simulink model "simulink_cordic_cart2pol_model"  (R2018a)
settings: Solver=FixedStepDiscrete  StartTime=0.0  StopTime=inf  RelTol=1e-3
undefined symbols (not defined in the file or in its folder): cordic_table, gap, niter, pipe, x_in, y_in
libraries: hdlsllib x3, simulink x2
settings Model: DataTypeOverride=Off  PauseTimes=42  Creator=cchung  LastModifiedBy=tbryan
settings DataIOCC: SaveOutput=off  SaveTime=off
settings OptimizationCC: BlockReduction=off  ConditionallyExecuteInputs=off  DefaultParameterBehavior=Inlined
settings DebuggingCC: AlgebraicLoopMsg=error  SingleTaskRateTransMsg=error
settings HardwareCC: ProdBitPerPointer=32  ProdBitPerSizeT=32  ProdBitPerPtrDiffT=32  ProdLargestAtomicFloat=None  ProdIntDivRoundTo=Undefined  ProdEndianess=Unspecified  ProdWordSize=32  ProdHWDeviceType=ASIC/FPGA->ASIC/FPGA  TargetBitPerLong=64  TargetBitPerPointer=64  TargetBitPerSizeT=64  TargetBitPerPtrDiffT=64  TargetLongLongMode=on  TargetIntDivRoundTo=Zero  TargetEndianess=LittleEndian  TargetWordSize=64  TargetHWDeviceType=Custom Processor->MATLAB Host Computer  ProdEqTarget=off

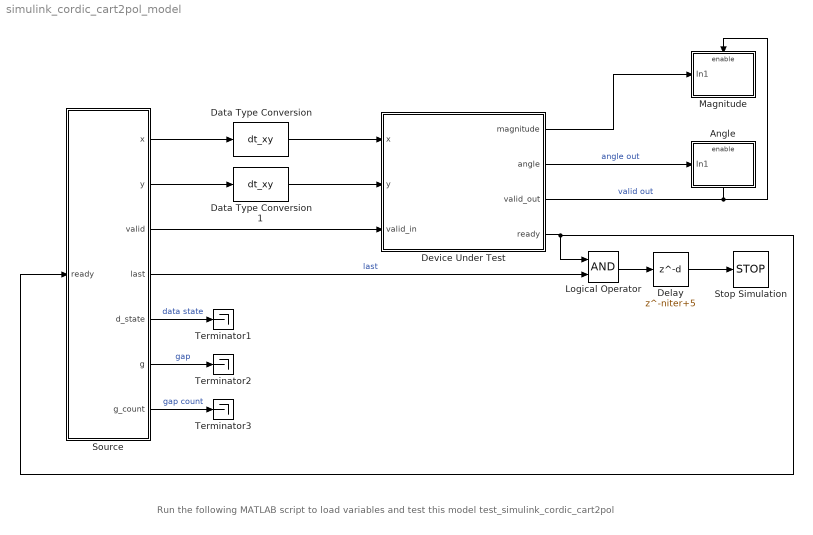
== system simulink_cordic_cart2pol_model ==
  note: Run the following MATLAB script to load variables and test this model
      | test_simulink_cordic_cart2pol
  Angle : Subsystem  TreatAsAtomicUnit=on
  Data Type Conversion : DataTypeConversion  OutDataTypeStr=dt_xy
  Data Type Conversion1 : DataTypeConversion  OutDataTypeStr=dt_xy
  Delay : Delay  DelayLength=niter+5
  Device Under Test : Subsystem
  Logical Operator : Logic  AllPortsSameDT=off  OutDataTypeStr=boolean
  Magnitude : Subsystem  TreatAsAtomicUnit=on
  Source : MATLAB Function  TreatAsAtomicUnit=on  SystemSampleTime=1
  Stop Simulation : Stop
  Terminator1 : Terminator
  Terminator2 : Terminator
  Terminator3 : Terminator
  wires:
  Device Under Test/2(angle) -> Angle/1(In1)  "angle out"
  Source/1(x) -> Data Type Conversion/1
  Source/2(y) -> Data Type Conversion1/1
  Data Type Conversion/1 -> Device Under Test/1(x)
  Data Type Conversion1/1 -> Device Under Test/2(y)
  Device Under Test/4(ready) -> Logical Operator/1, Source/1(ready)
  Source/3(valid) -> Device Under Test/3(valid_in)
  Source/4(last) -> Logical Operator/2  "last"
  Source/5(d_state) -> Terminator1/1  "data state"
  Source/6(g) -> Terminator2/1  "gap"
  Source/7(g_count) -> Terminator3/1  "gap count"
  Delay/1 -> Stop Simulation/1
  Logical Operator/1 -> Delay/1
  Device Under Test/1(magnitude) -> Magnitude/1(In1)
  Device Under Test/3(valid_out) -> Magnitude/Enable, Angle/Enable  "valid out"

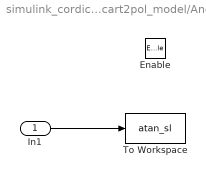
== system simulink_cordic_cart2pol_model/Angle ==
  In1 : Inport
  Enable : EnablePort
  To Workspace : ToWorkspace  VariableName=atan_sl  SampleTime=-1
      settings: Save2DSignal=2-D array (concatenate along first dimension)
  wires:
  In1/1 -> To Workspace/1

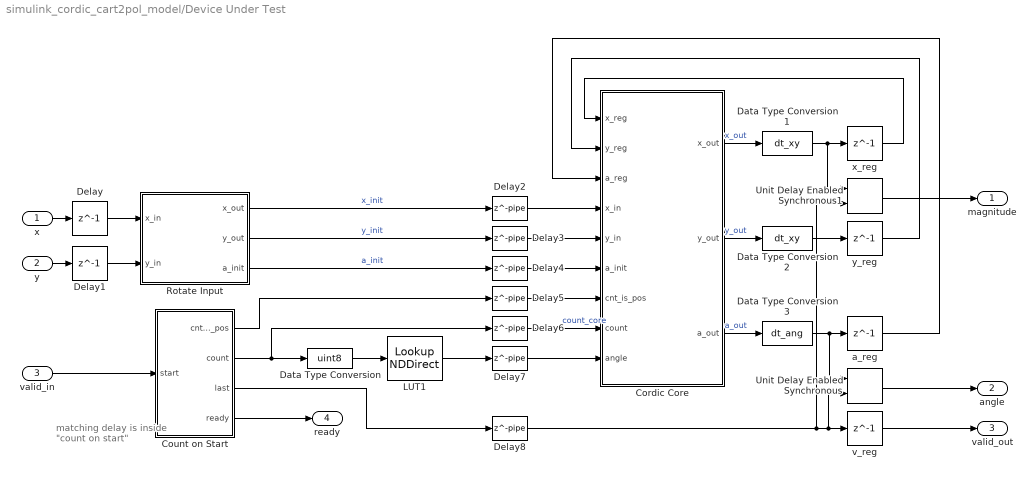
== system simulink_cordic_cart2pol_model/Device Under Test ==
  note: matching delay is
      | inside "count on start"
  x : Inport
  y : Inport  Port=2
  valid_in : Inport  Port=3
  Cordic Core : MATLAB Function  TreatAsAtomicUnit=on
  Count on Start : Subsystem  mask{cmax=niter-1}
      mask prompts: cmax "Count Max"
  Data Type Conversion : DataTypeConversion  OutDataTypeStr=uint8
  Data Type Conversion1 : DataTypeConversion  OutDataTypeStr=dt_xy
  Data Type Conversion2 : DataTypeConversion  OutDataTypeStr=dt_xy
  Data Type Conversion3 : DataTypeConversion  OutDataTypeStr=dt_ang
  Delay : Delay  DelayLength=1
  Delay1 : Delay  DelayLength=1
  Delay{2..8} (7 alike) : Delay  DelayLength=pipe
  LUT1 : LookupNDDirect  NumberOfTableDimensions=1  Table=cordic_table  DiagnosticForOutOfRangeInput=Error  TableDataTypeStr=dt_ang
  Rotate Input : MATLAB Function  TreatAsAtomicUnit=on
  Unit Delay Enabled Synchronous : hdlsllib/Discrete/Unit Delay Enabled Synchronous  InitialCondition=0.0  SampleTime=-1
      settings: SourceProductName=HDL Coder  SourceProductBaseCode=HD
  Unit Delay Enabled Synchronous1 : hdlsllib/Discrete/Unit Delay Enabled Synchronous  InitialCondition=0.0  SampleTime=-1
      settings: SourceProductName=HDL Coder  SourceProductBaseCode=HD
  a_reg : Delay  DelayLength=1
  v_reg : Delay  DelayLength=1
  x_reg : Delay  DelayLength=1
  y_reg : Delay  DelayLength=1
  magnitude : Outport
  angle : Outport  Port=2
  valid_out : Outport  Port=3
  ready : Outport  Port=4
  wires:
  y/1 -> Delay1/1
  x/1 -> Delay/1
  Rotate Input/1(x_out) -> Delay2/1  "x_init"
  Rotate Input/2(y_out) -> Delay3/1  "y_init"
  Rotate Input/3(a_init) -> Delay4/1  "a_init"
  Cordic Core/1(x_out) -> Data Type Conversion1/1  "x_out"
  Cordic Core/2(y_out) -> Data Type Conversion2/1  "y_out"
  Cordic Core/3(a_out) -> Data Type Conversion3/1  "a_out"
  x_reg/1 -> Cordic Core/1(x_reg)
  y_reg/1 -> Cordic Core/2(y_reg)
  a_reg/1 -> Cordic Core/3(a_reg)
  v_reg/1 -> valid_out/1
  Data Type Conversion1/1 -> Unit Delay Enabled Synchronous1/1, x_reg/1
  Data Type Conversion2/1 -> y_reg/1
  Data Type Conversion3/1 -> Unit Delay Enabled Synchronous/1, a_reg/1
  Delay/1 -> Rotate Input/1(x_in)
  Delay1/1 -> Rotate Input/2(y_in)
  valid_in/1 -> Count on Start/1(start)
  Count on Start/1(cnt_is_pos) -> Delay5/1
  Count on Start/2(count) -> Data Type Conversion/1, Delay6/1
  Count on Start/3(last) -> Delay8/1
  Count on Start/4(ready) -> ready/1
  Data Type Conversion/1 -> LUT1/1
  LUT1/1 -> Delay7/1
  Unit Delay Enabled Synchronous/1 -> angle/1
  Delay2/1 -> Cordic Core/4(x_in)
  Delay3/1 -> Cordic Core/5(y_in)
  Delay4/1 -> Cordic Core/6(a_init)
  Delay5/1 -> Cordic Core/7(cnt_is_pos)
  Delay6/1 -> Cordic Core/8(count)  "count_core"
  Delay7/1 -> Cordic Core/9(angle)
  Delay8/1 -> Unit Delay Enabled Synchronous1/2, Unit Delay Enabled Synchronous/2, v_reg/1
  Unit Delay Enabled Synchronous1/1 -> magnitude/1

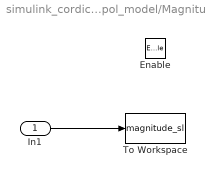
== system simulink_cordic_cart2pol_model/Magnitude ==
  In1 : Inport
  Enable : EnablePort
  To Workspace : ToWorkspace  VariableName=magnitude_sl  SampleTime=-1
      settings: Save2DSignal=2-D array (concatenate along first dimension)
  wires:
  In1/1 -> To Workspace/1

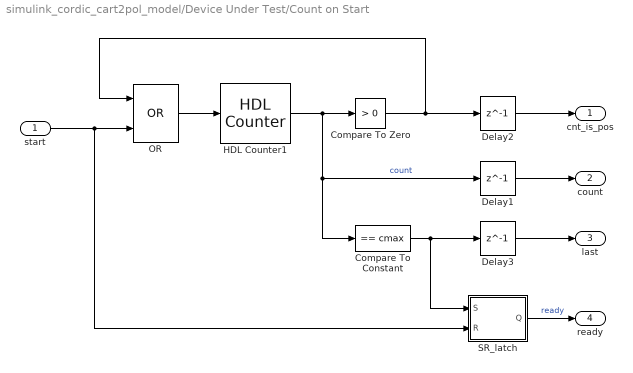
== system simulink_cordic_cart2pol_model/Device Under Test/Count on Start ==
  start : Inport
  Compare To Constant : simulink/Logic and Bit Operations/Compare To Constant  relop===  const=cmax  OutDataTypeStr=boolean
  Compare To Zero : simulink/Logic and Bit Operations/Compare To Zero  relop=>  OutDataTypeStr=boolean
  Delay1 : Delay  DelayLength=1
  Delay2 : Delay  DelayLength=1
  Delay3 : Delay  DelayLength=1
  HDL Counter1 : hdlsllib/Sources/HDL Counter  CountType=Count limited  CountInit=0  CountStep=1  CountMax=cmax  CountFromType=Initial value  CountFrom=0  CountResetPort=off  CountLoadPort=off  CountEnbPort=on  CountDirPort=off  CountDataType=Unsigned  CountWordLen=nextpow2(cmax+1)  CountFracLen=0  CountSampTime=1
      settings: SourceProductBaseCode=HD
  OR : Logic  Operator=OR  IconShape=distinctive  AllPortsSameDT=off  OutDataTypeStr=boolean
  SR_latch : Subsystem
  cnt_is_pos : Outport
  count : Outport  Port=2
  last : Outport  Port=3
  ready : Outport  Port=4
  wires:
  start/1 -> SR_latch/2(R), OR/2
  HDL Counter1/1 -> Compare To Zero/1, Compare To Constant/1, Delay1/1  "count"
  OR/1 -> HDL Counter1/1
  Compare To Zero/1 -> Delay2/1, OR/1
  Delay2/1 -> cnt_is_pos/1
  Delay1/1 -> count/1
  Delay3/1 -> last/1
  Compare To Constant/1 -> SR_latch/1(S), Delay3/1
  SR_latch/1(Q) -> ready/1  "ready"

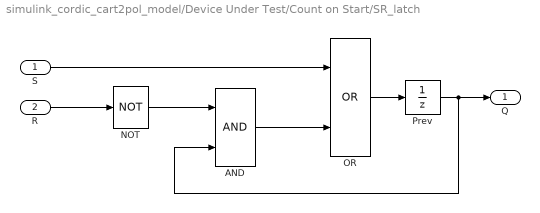
== system simulink_cordic_cart2pol_model/Device Under Test/Count on Start/SR_latch ==
  S : Inport
  R : Inport  Port=2
  AND : Logic  IconShape=distinctive  AllPortsSameDT=off  OutDataTypeStr=boolean
  NOT : Logic  Operator=NOT  IconShape=distinctive  AllPortsSameDT=off  OutDataTypeStr=boolean
  OR : Logic  Operator=OR  IconShape=distinctive  AllPortsSameDT=off  OutDataTypeStr=boolean
  Prev : UnitDelay  InitialCondition=1  SampleTime=-1
  Q : Outport
  wires:
  S/1 -> OR/1
  OR/1 -> Prev/1
  Prev/1 -> AND/2, Q/1
  AND/1 -> OR/2
  NOT/1 -> AND/1
  R/1 -> NOT/1

== matlab function simulink_cordic_cart2pol_model/Device Under Test/Rotate Input ==
  settings: fimath=hdlfimath
  data: x_in input; x_out output; y_in input; y_out output; a_init output; cordic_a0 parameter
function [x_out,y_out,a_init] = rotate_input(x_in,y_in,cordic_a0)
%#codegen
%
% Extracted from y5_atan_cr_rx_16Bit.m by Paul Voglewede 

% rotate the input signal between pi/2 and -pi/2
% use 90 degree method instead of 180 degree to avoid wrap issues
% add the performed rotation to the accumulated phase value

x_out = x_in;
y_out = y_in;
a_init = cast(0,'like',cordic_a0);

% not between pi/2 and -pi/2
if x_in < 0
    if y_in < 0  % rotate by +90 degrees
        x_out = -y_in;
        y_out =  x_in;
        a_init(:) = -bitsll(cordic_a0,1); 
    else % rotate by -90 degrees
        x_out =  y_in;
        y_out = -x_in;
        a_init(:) = bitsll(cordic_a0,1);
    end
end

== matlab function simulink_cordic_cart2pol_model/Device Under Test/Cordic Core ==
  settings: fimath=hdlfimath
  data: x_out output; y_out output; a_out output; x_reg input; y_reg input; a_reg input; x_in input; y_in input; a_init input; cnt_is_pos input; count input; angle input; wl_xy parameter
function [x_out,y_out,a_out] = cordic_core...
    (x_reg,y_reg,a_reg,x_in,y_in,a_init,cnt_is_pos,count,angle,wl_xy)
%#codegen
%
%   x(i+1) = x(i) - y(i)*d(i)*2^-i
%   y(i+1) = y(i) + x(i)*d(i)*2^-i
%   a(i+1) = a(i) - d(i)*atan(2^-i)
%
%       x(0) = real input sample
%       y(0) = imag input sample
%       a(0) = 0; angle of rotation
%       i = 0..N-1 ;  N is number of iterations
%       d(i) = +1 if y(i) < 0, else -1

% define data type
x_out = coder.nullcopy(x_in);
y_out = coder.nullcopy(y_in);
a_out = coder.nullcopy(a_init);

% intitialize the loop sum values
if cnt_is_pos
    x = x_reg;
    y = y_reg;
    a = a_reg;
else
    x = x_in;
    y = y_in;
    a = a_init;
end

%%%%%%%%%%%%%%%%%%%%%%%%%%%%%%%%%%
% first iteration
x_shifted = bitsra(x,count);
y_shifted = bitsra(y,count);

if bitget(y,wl_xy) == 0 % y1 >= 0
    % rotate the input vector
    x_out(:) = x + y_shifted;
    y_out(:) = y - x_shifted;
    % accumulate the phase being rotated
    a_out(:) = a + angle;
else
    x_out(:) = x - y_shifted;
    y_out(:) = y + x_shifted;
    a_out(:) = a - angle;
end

== matlab function simulink_cordic_cart2pol_model/Source ==
  data: ready input; x output; y output; x_in parameter; y_in parameter; gap parameter; valid output; last output; d_state output; g output; g_count output
function [x,y,valid,last,d_state,g,g_count] = fcn(ready,x_in,y_in,gap)

persistent data_state curr_gap gap_count samp_count; 
if isempty(data_state)
    data_state = 0;
    curr_gap = randi(gap);
    gap_count = 0;
    samp_count = 0;
end

% Debug only
d_state = data_state;
g = curr_gap;
g_count = gap_count;

if (samp_count == 0) || (samp_count > numel(x_in))
    valid = false;
    x = 0;
    y = 0;
else
    valid = (data_state > 0);
    x = x_in(samp_count);
    y = y_in(samp_count);
end

last = valid && (samp_count == numel(x_in));

switch data_state
    case 0 % wait for data
        if gap_count >= curr_gap
            data_state = 2;
        end
    case 1 % hold till ready
        if ready
            if curr_gap == 0
                data_state = 2; 
            else
                data_state = 0;
            end
        end            
    case 2 % send data
        if ready
            if curr_gap == 0
                data_state = 2;
            else
                data_state = 0;
            end
        else
            data_state = 1;
        end
end

if data_state == 2
    samp_count = samp_count + 1;
    gap_count = 0;
    curr_gap = randi(gap);
else
    gap_count = gap_count + 1;
end
